simulink model "czestotl"  (R2022b)
settings: Solver=VariableStepAuto  StartTime=0.0  StopTime=10  FixedStep=0.001  MaxStep=0.001  RelTol=1e-3
settings Model: Creator=zuzanna  LastModifiedBy=zuzanna

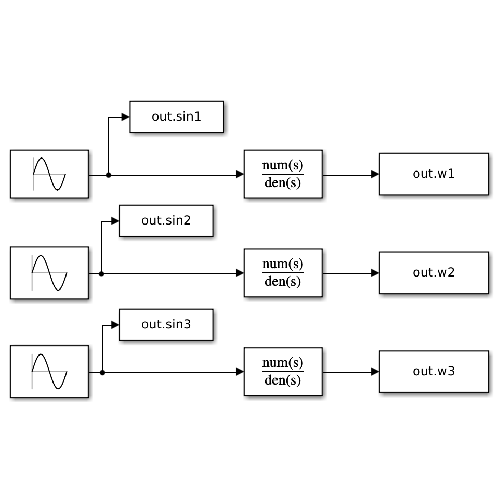
[thumbnail: Simulink's stored preview of the top-level diagram]
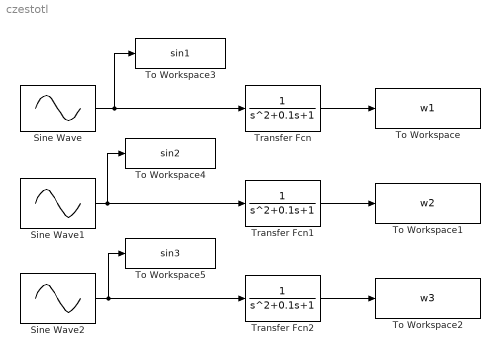
== system czestotl ==
  Sine Wave : Sin  Frequency=0.1  SampleTime=0
  Sine Wave1 : Sin  SampleTime=0
  Sine Wave2 : Sin  Frequency=10  SampleTime=0
  To Workspace : ToWorkspace  VariableName=w1  SampleTime=-1
      settings: Save2DSignal=2-D array (concatenate along first dimension)
  To Workspace1 : ToWorkspace  VariableName=w2  SampleTime=-1
      settings: Save2DSignal=2-D array (concatenate along first dimension)
  To Workspace2 : ToWorkspace  VariableName=w3  SampleTime=-1
      settings: Save2DSignal=2-D array (concatenate along first dimension)
  To Workspace3 : ToWorkspace  VariableName=sin1  SampleTime=-1
      settings: Save2DSignal=2-D array (concatenate along first dimension)
  To Workspace4 : ToWorkspace  VariableName=sin2  SampleTime=-1
      settings: Save2DSignal=2-D array (concatenate along first dimension)
  To Workspace5 : ToWorkspace  VariableName=sin3  SampleTime=-1
      settings: Save2DSignal=2-D array (concatenate along first dimension)
  Transfer Fcn : TransferFcn  Denominator=[1 0.1 1]
  Transfer Fcn1 : TransferFcn  Denominator=[1 0.1 1]
  Transfer Fcn2 : TransferFcn  Denominator=[1 0.1 1]
  wires:
  Transfer Fcn/1 -> To Workspace/1
  Sine Wave/1 -> To Workspace3/1, Transfer Fcn/1
  Transfer Fcn1/1 -> To Workspace1/1
  Sine Wave1/1 -> To Workspace4/1, Transfer Fcn1/1
  Transfer Fcn2/1 -> To Workspace2/1
  Sine Wave2/1 -> To Workspace5/1, Transfer Fcn2/1
